simulink model "Four_DG_MG_PrimaryOnly"  (R2021b)
settings: Solver=ode23tb  StartTime=0.0  StopTime=5  RelTol=1e-3
model workspace (MAT data in the model file):
  Ts : Simulink.Parameter (value not decoded)
  secondary_on : Simulink.Parameter (value not decoded)
values from neighbouring files (symbols this model uses):
  a12 = 0    [Four_DG_MG_PrimaryOnlyScript.m]    (also in MPC_MG_script_raw_dmpc.m; MPC_MG_secondary_script.m)
  a14 = 0    [Four_DG_MG_PrimaryOnlyScript.m]    (also in MPC_MG_script_raw_dmpc.m; MPC_MG_secondary_script.m)
  a21 = 1    [Four_DG_MG_PrimaryOnlyScript.m]    (also in MPC_MG_script_raw_dmpc.m; MPC_MG_secondary_script.m)
  a23 = 0    [Four_DG_MG_PrimaryOnlyScript.m]    (also in MPC_MG_script_raw_dmpc.m; MPC_MG_secondary_script.m)
  a32 = 1    [Four_DG_MG_PrimaryOnlyScript.m]    (also in MPC_MG_script_raw_dmpc.m; MPC_MG_secondary_script.m)
  a34 = 0    [Four_DG_MG_PrimaryOnlyScript.m]    (also in MPC_MG_script_raw_dmpc.m; MPC_MG_secondary_script.m)
  a41 = 1    [Four_DG_MG_PrimaryOnlyScript.m]    (also in MPC_MG_script_raw_dmpc.m; MPC_MG_secondary_script.m)
  a43 = 0    [Four_DG_MG_PrimaryOnlyScript.m]    (also in MPC_MG_script_raw_dmpc.m; MPC_MG_secondary_script.m)
  b1v = 1    [Four_DG_MG_PrimaryOnlyScript.m]    (also in MPC_MG_script_raw_dmpc.m; MPC_MG_secondary_script.m; MPG_MG_July.m; MPG_MG_freq_script.m)
  b1w = 1    [Four_DG_MG_PrimaryOnlyScript.m]    (also in MPC_MG_script_raw_dmpc.m; MPC_MG_secondary_script.m; MPG_MG_July.m; MPG_MG_freq_script.m)
  b2v = 0    [Four_DG_MG_PrimaryOnlyScript.m]    (also in MPC_MG_script_raw_dmpc.m; MPC_MG_secondary_script.m; MPG_MG_July.m; MPG_MG_freq_script.m)
  b2w = 0    [Four_DG_MG_PrimaryOnlyScript.m]    (also in MPC_MG_script_raw_dmpc.m; MPC_MG_secondary_script.m; MPG_MG_July.m; MPG_MG_freq_script.m)
  b3v = 0    [Four_DG_MG_PrimaryOnlyScript.m]    (also in MPC_MG_script_raw_dmpc.m; MPC_MG_secondary_script.m; MPG_MG_July.m; MPG_MG_freq_script.m)
  b3w = 0    [Four_DG_MG_PrimaryOnlyScript.m]    (also in MPC_MG_script_raw_dmpc.m; MPC_MG_secondary_script.m; MPG_MG_July.m; MPG_MG_freq_script.m)
  b4v = 0    [Four_DG_MG_PrimaryOnlyScript.m]    (also in MPC_MG_script_raw_dmpc.m; MPC_MG_secondary_script.m; MPG_MG_July.m; MPG_MG_freq_script.m)
  b4w = 0    [Four_DG_MG_PrimaryOnlyScript.m]    (also in MPC_MG_script_raw_dmpc.m; MPC_MG_secondary_script.m; MPG_MG_July.m; MPG_MG_freq_script.m)
  C_f = 50e-6    (= 5e-05)    [Four_DG_MG_PrimaryOnlyScript.m]    (also in MPC_MG_script.m; MPC_MG_script_raw_dmpc.m; MPC_MG_secondary_script.m; MPG_MG_July.m)
  cf = 60    [Four_DG_MG_PrimaryOnlyScript.m]    (also in MPC_MG_script_raw_dmpc.m = 40; MPC_MG_secondary_script.m = 40; MPG_MG_July.m = 100; MPG_MG_freq_script.m = 100)
  cv = 60    [Four_DG_MG_PrimaryOnlyScript.m]    (also in MPC_MG_script_raw_dmpc.m = 40; MPC_MG_secondary_script.m = 40; MPG_MG_July.m = 100; MPG_MG_freq_script.m = 100)
  F = 1    [Four_DG_MG_PrimaryOnlyScript.m]    (also in dmpc.m = zeros(9,1))
  K_i1 = 420    [Four_DG_MG_PrimaryOnlyScript.m]
  K_i2 = K_i1    (= 420)    [Four_DG_MG_PrimaryOnlyScript.m]
  K_i3 = 390    [Four_DG_MG_PrimaryOnlyScript.m]
  K_i4 = K_i3    (= 390)    [Four_DG_MG_PrimaryOnlyScript.m]
  K_ii1 = 5e3    (= 5000)    [Four_DG_MG_PrimaryOnlyScript.m]
  K_ii2 = K_ii1    (= 5000)    [Four_DG_MG_PrimaryOnlyScript.m]
  K_ii3 = 16e3    (= 16000)    [Four_DG_MG_PrimaryOnlyScript.m]
  K_ii4 = K_ii3    (= 16000)    [Four_DG_MG_PrimaryOnlyScript.m]
  K_p1 = 0.1    [Four_DG_MG_PrimaryOnlyScript.m]
  K_p2 = K_p1    (= 0.1)    [Four_DG_MG_PrimaryOnlyScript.m]
  K_p3 = 0.05    [Four_DG_MG_PrimaryOnlyScript.m]
  K_p4 = K_p3    (= 0.05)    [Four_DG_MG_PrimaryOnlyScript.m]
  K_pi1 = 5    [Four_DG_MG_PrimaryOnlyScript.m]
  K_pi2 = K_pi1    (= 5)    [Four_DG_MG_PrimaryOnlyScript.m]
  K_pi3 = 10.5    [Four_DG_MG_PrimaryOnlyScript.m]
  K_pi4 = K_pi3    (= 10.5)    [Four_DG_MG_PrimaryOnlyScript.m]
  L_f = 1.35e-3    (= 0.00135)    [Four_DG_MG_PrimaryOnlyScript.m]    (also in MPC_MG_script.m; MPC_MG_script_raw_dmpc.m; MPC_MG_secondary_script.m; MPG_MG_July.m)
  L_in1 = 0.35e-3    (= 0.00035)    [Four_DG_MG_PrimaryOnlyScript.m]    (also in MPC_MG_script.m; MPC_MG_script_raw_dmpc.m; MPC_MG_secondary_script.m; MPG_MG_July.m)
  L_in2 = 0.35e-3    (= 0.00035)    [Four_DG_MG_PrimaryOnlyScript.m]    (also in MPC_MG_script.m; MPC_MG_script_raw_dmpc.m; MPC_MG_secondary_script.m; MPG_MG_July.m)
  L_in3 = 0.35e-3    (= 0.00035)    [Four_DG_MG_PrimaryOnlyScript.m]    (also in MPC_MG_script.m; MPC_MG_script_raw_dmpc.m; MPC_MG_secondary_script.m; MPG_MG_July.m)
  L_in4 = 0.35e-3    (= 0.00035)    [Four_DG_MG_PrimaryOnlyScript.m]    (also in MPC_MG_script.m; MPC_MG_script_raw_dmpc.m; MPC_MG_secondary_script.m; MPG_MG_July.m)
  lo_co = 0.2    [Four_DG_MG_PrimaryOnlyScript.m]    (also in MPC_MG_script.m = 0.05; MPC_MG_script_raw_dmpc.m; MPC_MG_secondary_script.m = 0.08; MPG_MG_July.m = 0.15)
  m_p1 = 9.4e-5/droopDivide    (= 9.4e-05)    [Four_DG_MG_PrimaryOnlyScript.m]    (also in MPC_MG_script.m; MPC_MG_script_raw_dmpc.m; MPC_MG_secondary_script.m; MPG_MG_July.m)
  m_p2 = 9.4e-5/droopDivide    (= 9.4e-05)    [Four_DG_MG_PrimaryOnlyScript.m]    (also in MPC_MG_script.m; MPC_MG_script_raw_dmpc.m; MPC_MG_secondary_script.m; MPG_MG_July.m)
  m_p3 = 12.5e-5/droopDivide    (= 0.000125)    [Four_DG_MG_PrimaryOnlyScript.m]    (also in MPC_MG_script.m; MPC_MG_script_raw_dmpc.m; MPC_MG_secondary_script.m; MPG_MG_July.m)
  m_p4 = 12.5e-5/droopDivide    (= 0.000125)    [Four_DG_MG_PrimaryOnlyScript.m]    (also in MPC_MG_script.m; MPC_MG_script_raw_dmpc.m; MPC_MG_secondary_script.m; MPG_MG_July.m)
  n_q1 = 1.3e-3/droopDivide2    (= 0.00013)    [Four_DG_MG_PrimaryOnlyScript.m]    (also in MPC_MG_script.m; MPC_MG_script_raw_dmpc.m; MPC_MG_secondary_script.m; MPG_MG_July.m)
  n_q2 = 1.3e-3/droopDivide2    (= 0.00013)    [Four_DG_MG_PrimaryOnlyScript.m]    (also in MPC_MG_script.m; MPC_MG_script_raw_dmpc.m; MPC_MG_secondary_script.m; MPG_MG_July.m)
  n_q3 = 1.5e-3/droopDivide2    (= 0.00015)    [Four_DG_MG_PrimaryOnlyScript.m]    (also in MPC_MG_script.m; MPC_MG_script_raw_dmpc.m; MPC_MG_secondary_script.m; MPG_MG_July.m)
  n_q4 = 1.5e-3/droopDivide2    (= 0.00015)    [Four_DG_MG_PrimaryOnlyScript.m]    (also in MPC_MG_script.m; MPC_MG_script_raw_dmpc.m; MPC_MG_secondary_script.m; MPG_MG_July.m)
  pq_gain = 3/2    (= 1.5)    [Four_DG_MG_PrimaryOnlyScript.m]
  R_f = 0.1    [Four_DG_MG_PrimaryOnlyScript.m]    (also in MPC_MG_script.m; MPC_MG_script_raw_dmpc.m; MPC_MG_secondary_script.m; MPG_MG_July.m)
  R_in1 = 0.03    [Four_DG_MG_PrimaryOnlyScript.m]    (also in MPC_MG_script.m; MPC_MG_script_raw_dmpc.m; MPC_MG_secondary_script.m; MPG_MG_July.m)
  R_in2 = 0.03    [Four_DG_MG_PrimaryOnlyScript.m]    (also in MPC_MG_script.m; MPC_MG_script_raw_dmpc.m; MPC_MG_secondary_script.m; MPG_MG_July.m)
  R_in3 = 0.03    [Four_DG_MG_PrimaryOnlyScript.m]    (also in MPC_MG_script.m; MPC_MG_script_raw_dmpc.m; MPC_MG_secondary_script.m; MPG_MG_July.m)
  R_in4 = 0.03    [Four_DG_MG_PrimaryOnlyScript.m]    (also in MPC_MG_script.m; MPC_MG_script_raw_dmpc.m; MPC_MG_secondary_script.m; MPG_MG_July.m)
  secondary = 1    [Four_DG_MG_PrimaryOnlyScript.m]
  secondary2 = 1    [Four_DG_MG_PrimaryOnlyScript.m]
  time_thresh = 0.6    [Four_DG_MG_PrimaryOnlyScript.m]    (also in MPC_MG_script_raw_dmpc.m = 1.5; MPC_MG_secondary_script.m = 2; MPG_MG_July.m = 0.5; MPG_MG_freq_script.m = 0.5)
  Ts = 10e-6    (= 1e-05)    [Four_DG_MG_PrimaryOnlyScript.m]    (also in MPC_MG_script.m; MPC_MG_script_raw_dmpc.m; MPC_MG_secondary_script.m; MPG_MG_July.m)
  V_nom = 220*sqrt(2)    [Four_DG_MG_PrimaryOnlyScript.m]    (also in MPC_MG_script.m; MPC_MG_script_raw_dmpc.m; MPC_MG_secondary_script.m; MPG_MG_July.m)
  Vdc = 600    [Four_DG_MG_PrimaryOnlyScript.m]    (also in MPC_MG_script.m; MPC_MG_script_raw_dmpc.m; MPC_MG_secondary_script.m; MPG_MG_July.m)
  w_nom = 2*pi*50    (= 314.159265359)    [Four_DG_MG_PrimaryOnlyScript.m]    (also in MPC_MG_script.m; MPC_MG_script_raw_dmpc.m; MPC_MG_secondary_script.m; MPG_MG_July.m)
undefined symbols (not defined in the file or in its folder): K_d
libraries: slpidlib x16, spsThreePhaseSeriesRLCBranchLib x15, spsabctodq0Lib x13, spsThreePhaseVIMeasurementLib x12, eeGeneralControl x8, spsOnDelayLib x8, spsPMUPLLBasedPositiveSequenceLib x4, eePwmGeneratorTwoLevel x4, spsdq0toabcLib x4, spsDCVoltageSourceLib x4, spsSeriesRLCBranchLib x4, spsTwoLevelConverterLib x4
(part 3 of 4)

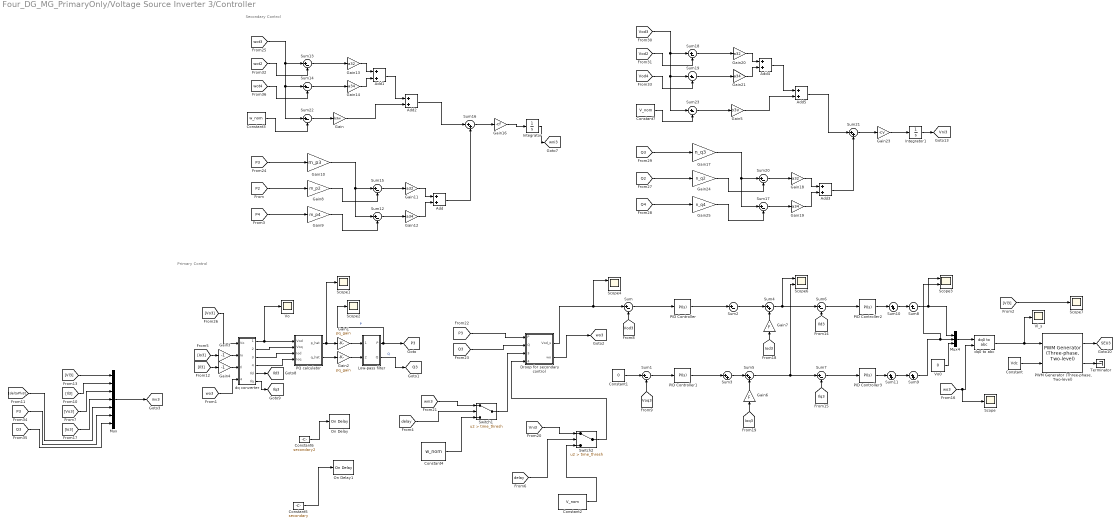
== system Four_DG_MG_PrimaryOnly/Voltage Source Inverter 3/Controller ==
  note: Secondary Control
  note: Primary Control
  Add{,1..5} (6 alike) : Sum
  Constant : Constant  Value=Vdc
  Constant1 : Constant  Value=0
  Constant2 : Constant  Value=V_nom
  Constant3 : Constant  Value=w_nom
  Constant4 : Constant  Value=w_nom
  Constant5 : Constant  Value=secondary
  Constant6 : Constant  Value=secondary2
  Constant7 : Constant  Value=V_nom
  Droop for secondary control : Subsystem
  Gain : Gain  Gain=b3w
  Gain1 : Gain  Gain=pq_gain
  Gain10 : Gain  Gain=m_p3
  Gain{11,13,18,20} (4 alike) : Gain  Gain=a32
  Gain{12,14,19,21} (4 alike) : Gain  Gain=a34
  Gain16 : Gain  Gain=-cf
  Gain17 : Gain  Gain=n_q3
  Gain2 : Gain  Gain=pq_gain
  Gain23 : Gain  Gain=-cv
  Gain24 : Gain  Gain=n_q2
  Gain25 : Gain  Gain=n_q4
  Gain3 : Gain  Gain=-1
  Gain4 : Gain  Gain=-1
  Gain5 : Gain  Gain=b3v
  Gain6 : Gain  Gain=F
  Gain7 : Gain  Gain=F
  Gain8 : Gain  Gain=m_p2
  Gain9 : Gain  Gain=m_p4
  Integrator : Integrator  InitialCondition=50*2*pi  UpperSaturationLimit=51*2*pi  LowerSaturationLimit=50*2*pi
  Integrator1 : Integrator  InitialCondition=311  UpperSaturationLimit=373.35  LowerSaturationLimit=248.90
  Low-pass filter : Subsystem
  Mux : Mux  Inputs=7
  Mux4 : Mux  Inputs=3
  On Delay : spsOnDelayLib/On Delay  DelayType=On delay  delay=4  ic=0  Ts=0
      settings: SourceProductBaseCode=PS
  On Delay1 : spsOnDelayLib/On Delay  DelayType=On delay  delay=4  ic=0  Ts=0
      settings: SourceProductBaseCode=PS
  PID Controller : slpidlib/PID Controller  Controller=PI  Form=Parallel  TimeDomain=Continuous-time  UseExternalTs=off  SampleTime=-1  IntegratorMethod=Forward Euler  FilterMethod=Forward Euler  ControllerParametersSource=internal  P=K_p3  I=K_i3  D=K_d  UseFilter=on  N=100  TunerSelectOption=Frequency Response Based  InitialConditionSource=internal  InitialConditionForIntegrator=0  InitialConditionForFilter=0  DifferentiatorICPrevScaledInput=0  ExternalReset=none  TrackingMode=off  Kt=1  LimitOutput=off  SatLimitsSource=internal  UpperSaturationLimit=50  LowerSaturationLimit=-50  LinearizeAsGain=on  AntiWindupMode=none  Kb=1  POutMin=[]  POutMax=[]  IOutMin=[]  IOutMax=[]  DOutMin=[]  DOutMax=[]  NOutMin=[]  NOutMax=[]  SumOutMin=[]  SumOutMax=[]  SaturationOutMin=[]  SaturationOutMax=[]  PParamMin=[]  PParamMax=[]  IParamMin=[]  IParamMax=[]  DParamMin=[]  DParamMax=[]  NParamMin=[]  NParamMax=[]  KbParamMin=[]  KbParamMax=[]  KtParamMin=[]  KtParamMax=[]  KbOutMin=[]  KbOutMax=[]  KtOutMin=[]  KtOutMax=[]  IntegratorOutMin=[]  IntegratorOutMax=[]  FilterOutMin=[]  FilterOutMax=[]  SumI1OutMin=[]  SumI1OutMax=[]  SumI2OutMin=[]  SumI2OutMax=[]  SumI3OutMin=[]  SumI3OutMax=[]  SumI4OutMin=[]  SumI4OutMax=[]  SumDOutMin=[]  SumDOutMax=[]  DifferentiatorOutMin=[]  DifferentiatorOutMax=[]  FilterDiffOutCoefMin=[]  FilterDiffOutCoefMax=[]  ReciprocalOutMin=[]  ReciprocalOutMax=[]  SumDenOutMin=[]  SumDenOutMax=[]  SumNumOutMin=[]  SumNumOutMax=[]  DivideOutMin=[]  DivideOutMax=[]  UdiffTsProdOutMin=[]  UdiffTsProdOutMax=[]  NTsProdOutMin=[]  NTsProdOutMax=[]  UintegralTsProdOutMin=[]  UintegralTsProdOutMax=[]  UngainTsProdOutMin=[]  UngainTsProdOutMax=[]  IntegratorContinuousStateAttributes=''  IntegratorStateMustResolveToSignalObject=off  IntegratorRTWStateStorageClass=Auto  FilterContinuousStateAttributes=''  FilterStateMustResolveToSignalObject=off  FilterRTWStateStorageClass=Auto  ParallelPVariant=InternalParameters  IdealPVariant=Disabled  IVariant=InternalParameters  DVariant=Disabled  IntegratorVariant=Continuous  SatVariant=Disabled  AWVariant=Passthrough  PCopyVariant=Disabled  TRVariant=Disabled  FdbkBlocksVariant=Forward  IdealPFdbkVariant=Disabled  SatFdbkVariant=Disabled  DerivativeFilterVariant=Disabled  NVariant=Disabled  NCopyVariant=Disabled_SignalSpec  FilterICVariant=Disabled  IntegratorICVariant=InternalICs  ExternalResetVariant=Disabled  TRSumVariant=Passthrough  SumFdbkVariant=Disabled  SumVariant=Sum_PI  TsampFilterVariant=InternalTs  TsampNgainVariant=Passthrough  TsampIntegralVariant=Passthrough  ExternalSaturationOutDataTypeStr=Inherit: Same as second input
  PID Controller1 : slpidlib/PID Controller  Controller=PI  Form=Parallel  TimeDomain=Continuous-time  UseExternalTs=off  SampleTime=-1  IntegratorMethod=Forward Euler  FilterMethod=Forward Euler  ControllerParametersSource=internal  P=K_p3  I=K_i3  D=K_d  UseFilter=on  N=100  TunerSelectOption=Frequency Response Based  InitialConditionSource=internal  InitialConditionForIntegrator=0  InitialConditionForFilter=0  DifferentiatorICPrevScaledInput=0  ExternalReset=none  TrackingMode=off  Kt=1  LimitOutput=off  SatLimitsSource=internal  UpperSaturationLimit=50  LowerSaturationLimit=-50  LinearizeAsGain=on  AntiWindupMode=none  Kb=1  POutMin=[]  POutMax=[]  IOutMin=[]  IOutMax=[]  DOutMin=[]  DOutMax=[]  NOutMin=[]  NOutMax=[]  SumOutMin=[]  SumOutMax=[]  SaturationOutMin=[]  SaturationOutMax=[]  PParamMin=[]  PParamMax=[]  IParamMin=[]  IParamMax=[]  DParamMin=[]  DParamMax=[]  NParamMin=[]  NParamMax=[]  KbParamMin=[]  KbParamMax=[]  KtParamMin=[]  KtParamMax=[]  KbOutMin=[]  KbOutMax=[]  KtOutMin=[]  KtOutMax=[]  IntegratorOutMin=[]  IntegratorOutMax=[]  FilterOutMin=[]  FilterOutMax=[]  SumI1OutMin=[]  SumI1OutMax=[]  SumI2OutMin=[]  SumI2OutMax=[]  SumI3OutMin=[]  SumI3OutMax=[]  SumI4OutMin=[]  SumI4OutMax=[]  SumDOutMin=[]  SumDOutMax=[]  DifferentiatorOutMin=[]  DifferentiatorOutMax=[]  FilterDiffOutCoefMin=[]  FilterDiffOutCoefMax=[]  ReciprocalOutMin=[]  ReciprocalOutMax=[]  SumDenOutMin=[]  SumDenOutMax=[]  SumNumOutMin=[]  SumNumOutMax=[]  DivideOutMin=[]  DivideOutMax=[]  UdiffTsProdOutMin=[]  UdiffTsProdOutMax=[]  NTsProdOutMin=[]  NTsProdOutMax=[]  UintegralTsProdOutMin=[]  UintegralTsProdOutMax=[]  UngainTsProdOutMin=[]  UngainTsProdOutMax=[]  IntegratorContinuousStateAttributes=''  IntegratorStateMustResolveToSignalObject=off  IntegratorRTWStateStorageClass=Auto  FilterContinuousStateAttributes=''  FilterStateMustResolveToSignalObject=off  FilterRTWStateStorageClass=Auto  ParallelPVariant=InternalParameters  IdealPVariant=Disabled  IVariant=InternalParameters  DVariant=Disabled  IntegratorVariant=Continuous  SatVariant=Disabled  AWVariant=Passthrough  PCopyVariant=Disabled  TRVariant=Disabled  FdbkBlocksVariant=Forward  IdealPFdbkVariant=Disabled  SatFdbkVariant=Disabled  DerivativeFilterVariant=Disabled  NVariant=Disabled  NCopyVariant=Disabled_SignalSpec  FilterICVariant=Disabled  IntegratorICVariant=InternalICs  ExternalResetVariant=Disabled  TRSumVariant=Passthrough  SumFdbkVariant=Disabled  SumVariant=Sum_PI  TsampFilterVariant=InternalTs  TsampNgainVariant=Passthrough  TsampIntegralVariant=Passthrough  ExternalSaturationOutDataTypeStr=Inherit: Same as second input
  PID Controller2 : slpidlib/PID Controller  Controller=PI  Form=Parallel  TimeDomain=Continuous-time  UseExternalTs=off  SampleTime=-1  IntegratorMethod=Forward Euler  FilterMethod=Forward Euler  ControllerParametersSource=internal  P=K_pi3  I=K_ii3  D=K_d  UseFilter=on  N=100  TunerSelectOption=Frequency Response Based  InitialConditionSource=internal  InitialConditionForIntegrator=0  InitialConditionForFilter=0  DifferentiatorICPrevScaledInput=0  ExternalReset=none  TrackingMode=off  Kt=1  LimitOutput=off  SatLimitsSource=internal  UpperSaturationLimit=inf  LowerSaturationLimit=-inf  LinearizeAsGain=on  AntiWindupMode=none  Kb=1  POutMin=[]  POutMax=[]  IOutMin=[]  IOutMax=[]  DOutMin=[]  DOutMax=[]  NOutMin=[]  NOutMax=[]  SumOutMin=[]  SumOutMax=[]  SaturationOutMin=[]  SaturationOutMax=[]  PParamMin=[]  PParamMax=[]  IParamMin=[]  IParamMax=[]  DParamMin=[]  DParamMax=[]  NParamMin=[]  NParamMax=[]  KbParamMin=[]  KbParamMax=[]  KtParamMin=[]  KtParamMax=[]  KbOutMin=[]  KbOutMax=[]  KtOutMin=[]  KtOutMax=[]  IntegratorOutMin=[]  IntegratorOutMax=[]  FilterOutMin=[]  FilterOutMax=[]  SumI1OutMin=[]  SumI1OutMax=[]  SumI2OutMin=[]  SumI2OutMax=[]  SumI3OutMin=[]  SumI3OutMax=[]  SumI4OutMin=[]  SumI4OutMax=[]  SumDOutMin=[]  SumDOutMax=[]  DifferentiatorOutMin=[]  DifferentiatorOutMax=[]  FilterDiffOutCoefMin=[]  FilterDiffOutCoefMax=[]  ReciprocalOutMin=[]  ReciprocalOutMax=[]  SumDenOutMin=[]  SumDenOutMax=[]  SumNumOutMin=[]  SumNumOutMax=[]  DivideOutMin=[]  DivideOutMax=[]  UdiffTsProdOutMin=[]  UdiffTsProdOutMax=[]  NTsProdOutMin=[]  NTsProdOutMax=[]  UintegralTsProdOutMin=[]  UintegralTsProdOutMax=[]  UngainTsProdOutMin=[]  UngainTsProdOutMax=[]  IntegratorContinuousStateAttributes=''  IntegratorStateMustResolveToSignalObject=off  IntegratorRTWStateStorageClass=Auto  FilterContinuousStateAttributes=''  FilterStateMustResolveToSignalObject=off  FilterRTWStateStorageClass=Auto  ParallelPVariant=InternalParameters  IdealPVariant=Disabled  IVariant=InternalParameters  DVariant=Disabled  IntegratorVariant=Continuous  SatVariant=Disabled  AWVariant=Passthrough  PCopyVariant=Disabled  TRVariant=Disabled  FdbkBlocksVariant=Forward  IdealPFdbkVariant=Disabled  SatFdbkVariant=Disabled  DerivativeFilterVariant=Disabled  NVariant=Disabled  NCopyVariant=Disabled_SignalSpec  FilterICVariant=Disabled  IntegratorICVariant=InternalICs  ExternalResetVariant=Disabled  TRSumVariant=Passthrough  SumFdbkVariant=Disabled  SumVariant=Sum_PI  TsampFilterVariant=InternalTs  TsampNgainVariant=Passthrough  TsampIntegralVariant=Passthrough  ExternalSaturationOutDataTypeStr=Inherit: Same as second input
  PID Controller3 : slpidlib/PID Controller  Controller=PI  Form=Parallel  TimeDomain=Continuous-time  UseExternalTs=off  SampleTime=-1  IntegratorMethod=Forward Euler  FilterMethod=Forward Euler  ControllerParametersSource=internal  P=K_pi3  I=K_ii3  D=K_d  UseFilter=on  N=100  TunerSelectOption=Frequency Response Based  InitialConditionSource=internal  InitialConditionForIntegrator=0  InitialConditionForFilter=0  DifferentiatorICPrevScaledInput=0  ExternalReset=none  TrackingMode=off  Kt=1  LimitOutput=off  SatLimitsSource=internal  UpperSaturationLimit=inf  LowerSaturationLimit=-inf  LinearizeAsGain=on  AntiWindupMode=none  Kb=1  POutMin=[]  POutMax=[]  IOutMin=[]  IOutMax=[]  DOutMin=[]  DOutMax=[]  NOutMin=[]  NOutMax=[]  SumOutMin=[]  SumOutMax=[]  SaturationOutMin=[]  SaturationOutMax=[]  PParamMin=[]  PParamMax=[]  IParamMin=[]  IParamMax=[]  DParamMin=[]  DParamMax=[]  NParamMin=[]  NParamMax=[]  KbParamMin=[]  KbParamMax=[]  KtParamMin=[]  KtParamMax=[]  KbOutMin=[]  KbOutMax=[]  KtOutMin=[]  KtOutMax=[]  IntegratorOutMin=[]  IntegratorOutMax=[]  FilterOutMin=[]  FilterOutMax=[]  SumI1OutMin=[]  SumI1OutMax=[]  SumI2OutMin=[]  SumI2OutMax=[]  SumI3OutMin=[]  SumI3OutMax=[]  SumI4OutMin=[]  SumI4OutMax=[]  SumDOutMin=[]  SumDOutMax=[]  DifferentiatorOutMin=[]  DifferentiatorOutMax=[]  FilterDiffOutCoefMin=[]  FilterDiffOutCoefMax=[]  ReciprocalOutMin=[]  ReciprocalOutMax=[]  SumDenOutMin=[]  SumDenOutMax=[]  SumNumOutMin=[]  SumNumOutMax=[]  DivideOutMin=[]  DivideOutMax=[]  UdiffTsProdOutMin=[]  UdiffTsProdOutMax=[]  NTsProdOutMin=[]  NTsProdOutMax=[]  UintegralTsProdOutMin=[]  UintegralTsProdOutMax=[]  UngainTsProdOutMin=[]  UngainTsProdOutMax=[]  IntegratorContinuousStateAttributes=''  IntegratorStateMustResolveToSignalObject=off  IntegratorRTWStateStorageClass=Auto  FilterContinuousStateAttributes=''  FilterStateMustResolveToSignalObject=off  FilterRTWStateStorageClass=Auto  ParallelPVariant=InternalParameters  IdealPVariant=Disabled  IVariant=InternalParameters  DVariant=Disabled  IntegratorVariant=Continuous  SatVariant=Disabled  AWVariant=Passthrough  PCopyVariant=Disabled  TRVariant=Disabled  FdbkBlocksVariant=Forward  IdealPFdbkVariant=Disabled  SatFdbkVariant=Disabled  DerivativeFilterVariant=Disabled  NVariant=Disabled  NCopyVariant=Disabled_SignalSpec  FilterICVariant=Disabled  IntegratorICVariant=InternalICs  ExternalResetVariant=Disabled  TRSumVariant=Passthrough  SumFdbkVariant=Disabled  SumVariant=Sum_PI  TsampFilterVariant=InternalTs  TsampNgainVariant=Passthrough  TsampIntegralVariant=Passthrough  ExternalSaturationOutDataTypeStr=Inherit: Same as second input
  PQ calculator : Subsystem
  "PWM Generator (Three-phase, Two-level)" : eePwmGeneratorTwoLevel/PWM Generator (Three-phase, Two-level)  PWMMode=Continuous PWM (CPWM)  CPWMMode=SPWM: sinusoidal PWM  DPWMMode=60 DPWM: 60 degree discontinuous PWM  fsw=f_c  Ts=Ts
      settings: SourceProductBaseCode=PS
  Scope{,1..2,7} (4 alike) : Scope
  Scope3 : Scope  NumInputPorts=2
  Scope4 : Scope  NumInputPorts=2
  Scope6 : Scope  NumInputPorts=2
  Sum{,1..2,6..8,12..15,17..20,22..23} (16 alike) : Sum  Inputs=|+-
  Sum{3..5,9..11,16,21} (8 alike) : Sum  Inputs=|++
  Switch1 : Switch  Criteria=u2 > Threshold  Threshold=time_thresh
  Switch2 : Switch  Criteria=u2 > Threshold  Threshold=time_thresh
  Terminator : Terminator
  Vl_s : Scope
  Vo : Scope
  Vo0 : Constant  Value=0
  dq converter : Subsystem
  dq0 to abc : spsdq0toabcLib/dq0 to abc  Alignment=90 degrees behind phase A axis
  tag scope: Ild3=global, Ilq3=global, P3=global, Q3=global, SEU3=global, Vni3=global, inv3=global, wni3=global, wo3=global
  wires:
  dq converter/1(Vod) -> Vo/1, PQ calculator/1(Vod)
  ? -> Sum3/2
  [Vl3] -> Scope7/1
  [Io3] -> Gain3/1
  Sum/1 -> PID Controller/1
  dq converter/6(Ilq) -> [Ilq3]
  Sum1/1 -> PID Controller1/1
  Sum7/1 -> PID Controller3/1
  [Voq3] -> Sum1/2
  dq converter/5(Ild) -> [Ild3]
  Mux4/1 -> dq0 to abc/1
  PID Controller/1 -> Sum2/1
  PID Controller1/1 -> Sum3/1
  Vo0/1 -> Mux4/3
  Sum6/1 -> PID Controller2/1
  Sum2/1 -> Sum4/1
  PQ calculator/1(p_hat) -> Gain1/1, Scope1/1
  [Il3] -> Gain4/1
  [Vo3] -> dq converter/1(Vo)
  Sum9/1 -> Scope3/2, Mux4/2
  Gain6/1 -> Sum5/2
  dq converter/4(Ioq) -> PQ calculator/4(Ioq)
  "PWM Generator (Three-phase, Two-level)"/2 -> Terminator/1
  Sum5/1 -> Scope6/2, Sum7/1
  Constant/1 -> "PWM Generator (Three-phase, Two-level)"/2
  dq converter/3(Iod) -> PQ calculator/3(Iod)
  dq converter/2(Voq) -> PQ calculator/2(Voq)
  Sum8/1 -> Scope3/1, Mux4/1
  [Ioq3] -> Gain6/1
  dq0 to abc/1 -> Vl_s/1, "PWM Generator (Three-phase, Two-level)"/1
  [Ilq3] -> Sum7/2
  Gain1/1 -> Low-pass filter/1(p_hat)
  "PWM Generator (Three-phase, Two-level)"/1 -> [SEU3]
  [Ild3] -> Sum6/2
  [Vod3] -> Sum/2
  PQ calculator/2(q_hat) -> Gain2/1
  Low-pass filter/1(P) -> [P3], Scope2/1  "P"
  Droop for secondary control/2(wo) -> [wo3]
  [Q3] -> Droop for secondary control/2(Q)
  [P3] -> Droop for secondary control/1(P)
  Gain7/1 -> Sum4/2
  [Iod3] -> Gain7/1
  Sum4/1 -> Scope6/1, Sum6/1
  Sum3/1 -> Sum5/1
  Gain2/1 -> Low-pass filter/2(q_hat)
  Low-pass filter/2(Q) -> [Q3]  "Q"
  [wni3] -> Switch1/1
  Constant4/1 -> Switch1/3
  Switch1/1 -> Droop for secondary control/3(w_nom)
  Switch2/1 -> Droop for secondary control/4(V_nom)
  [Vni3] -> Switch2/1
  Constant2/1 -> Switch2/3
  [wo3] -> Scope/1, dq0 to abc/2
  [wo3] -> dq converter/4(wo3)
  Droop for secondary control/1(Vod_s) -> Scope4/1, Sum/1
  PID Controller3/1 -> Sum11/1
  Sum11/1 -> Sum9/1
  PID Controller2/1 -> Sum10/1
  Sum10/1 -> Sum8/1
  Constant1/1 -> Sum1/1
  Gain3/1 -> dq converter/2(Io)
  Gain4/1 -> dq converter/3(Il)
  Sum16/1 -> Gain16/1
  [Q2] -> Gain24/1
  Gain10/1 -> Sum12/1, Sum15/1
  Sum14/1 -> Gain14/1
  [wot2] -> Sum13/2
  Integrator/1 -> [wni3]
  Gain13/1 -> Add1/1
  Gain19/1 -> Add3/2
  [Vod4] -> Sum19/2
  Sum17/1 -> Gain19/1
  [Q3] -> Gain17/1
  Sum21/1 -> Gain23/1
  [Vod3] -> Sum23/1, Sum19/1, Sum18/1
  Gain9/1 -> Sum12/2
  Gain24/1 -> Sum20/2
  Gain11/1 -> Add/1
  [P4] -> Gain9/1
  Sum13/1 -> Gain13/1
  Sum20/1 -> Gain18/1
  [Q4] -> Gain25/1
  Sum12/1 -> Gain12/1
  Gain16/1 -> Integrator/1
  Gain8/1 -> Sum15/2
  Gain25/1 -> Sum17/2
  Sum15/1 -> Gain11/1
  Add3/1 -> Sum21/2
  Gain14/1 -> Add1/2
  Sum19/1 -> Gain21/1
  [wot4] -> Sum14/2
  Gain21/1 -> Add4/2
  Add/1 -> Sum16/2
  [wot3] -> Sum22/1, Sum14/1, Sum13/1
  [Vod2] -> Sum18/2
  Gain20/1 -> Add4/1
  Integrator1/1 -> [Vni3]
  Gain12/1 -> Add/2
  Gain18/1 -> Add3/1
  Sum18/1 -> Gain20/1
  Gain17/1 -> Sum17/1, Sum20/1
  [P3] -> Gain10/1
  Gain23/1 -> Integrator1/1
  [P2] -> Gain8/1
  Constant6/1 -> On Delay/1
  Constant5/1 -> On Delay1/1
  [delay] -> Switch1/2
  [delay] -> Switch2/2
  Constant3/1 -> Sum22/2
  Sum22/1 -> Gain/1
  Add1/1 -> Add2/1
  Gain/1 -> Add2/2
  Add2/1 -> Sum16/1
  Constant7/1 -> Sum23/2
  Sum23/1 -> Gain5/1
  Add4/1 -> Add5/1
  Gain5/1 -> Add5/2
  Add5/1 -> Sum21/1
  [Vo3] -> Mux/3
  [P3] -> Mux/6
  [deltaPhi3] -> Mux/5
  [Vl3] -> Mux/1
  Mux/1 -> [inv3]
  [Q3] -> Mux/7
  [Il3] -> Mux/2
  [Io3] -> Mux/4

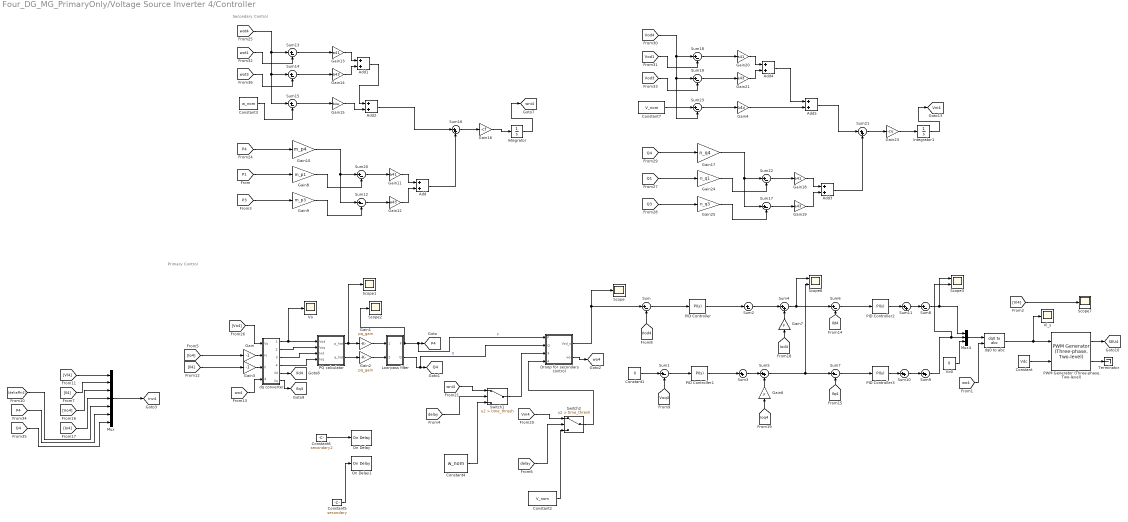
== system Four_DG_MG_PrimaryOnly/Voltage Source Inverter 4/Controller ==
  note: Secondary Control
  note: Primary Control
  Add{,1..5} (6 alike) : Sum
  Constant : Constant  Value=Vdc
  Constant1 : Constant  Value=0
  Constant2 : Constant  Value=V_nom
  Constant3 : Constant  Value=w_nom
  Constant4 : Constant  Value=w_nom
  Constant5 : Constant  Value=secondary
  Constant6 : Constant  Value=secondary2
  Constant7 : Constant  Value=V_nom
  Droop for secondary control : Subsystem
  Gain : Gain  Gain=-1
  Gain1 : Gain  Gain=pq_gain
  Gain10 : Gain  Gain=m_p4
  Gain{11,13,18,20} (4 alike) : Gain  Gain=a41
  Gain{12,14,19,21} (4 alike) : Gain  Gain=a43
  Gain15 : Gain  Gain=b4w
  Gain16 : Gain  Gain=-cf
  Gain17 : Gain  Gain=n_q4
  Gain2 : Gain  Gain=pq_gain
  Gain23 : Gain  Gain=-cv
  Gain24 : Gain  Gain=n_q1
  Gain25 : Gain  Gain=n_q3
  Gain3 : Gain  Gain=-1
  Gain4 : Gain  Gain=b4v
  Gain6 : Gain  Gain=F
  Gain7 : Gain  Gain=F
  Gain8 : Gain  Gain=m_p1
  Gain9 : Gain  Gain=m_p3
  Integrator : Integrator  InitialCondition=50*2*pi  UpperSaturationLimit=51*2*pi  LowerSaturationLimit=50*2*pi
  Integrator1 : Integrator  InitialCondition=311  UpperSaturationLimit=373.35  LowerSaturationLimit=248.90
  Low-pass filter : Subsystem
  Mux : Mux  Inputs=7
  Mux4 : Mux  Inputs=3
  On Delay : spsOnDelayLib/On Delay  DelayType=On delay  delay=4  ic=0  Ts=0
      settings: SourceProductBaseCode=PS
  On Delay1 : spsOnDelayLib/On Delay  DelayType=On delay  delay=4  ic=0  Ts=0
      settings: SourceProductBaseCode=PS
  PID Controller : slpidlib/PID Controller  Controller=PI  Form=Parallel  TimeDomain=Continuous-time  UseExternalTs=off  SampleTime=-1  IntegratorMethod=Forward Euler  FilterMethod=Forward Euler  ControllerParametersSource=internal  P=K_p4  I=K_i4  D=K_d  UseFilter=on  N=100  TunerSelectOption=Frequency Response Based  InitialConditionSource=internal  InitialConditionForIntegrator=0  InitialConditionForFilter=0  DifferentiatorICPrevScaledInput=0  ExternalReset=none  TrackingMode=off  Kt=1  LimitOutput=off  SatLimitsSource=internal  UpperSaturationLimit=50  LowerSaturationLimit=-50  LinearizeAsGain=on  AntiWindupMode=none  Kb=1  POutMin=[]  POutMax=[]  IOutMin=[]  IOutMax=[]  DOutMin=[]  DOutMax=[]  NOutMin=[]  NOutMax=[]  SumOutMin=[]  SumOutMax=[]  SaturationOutMin=[]  SaturationOutMax=[]  PParamMin=[]  PParamMax=[]  IParamMin=[]  IParamMax=[]  DParamMin=[]  DParamMax=[]  NParamMin=[]  NParamMax=[]  KbParamMin=[]  KbParamMax=[]  KtParamMin=[]  KtParamMax=[]  KbOutMin=[]  KbOutMax=[]  KtOutMin=[]  KtOutMax=[]  IntegratorOutMin=[]  IntegratorOutMax=[]  FilterOutMin=[]  FilterOutMax=[]  SumI1OutMin=[]  SumI1OutMax=[]  SumI2OutMin=[]  SumI2OutMax=[]  SumI3OutMin=[]  SumI3OutMax=[]  SumI4OutMin=[]  SumI4OutMax=[]  SumDOutMin=[]  SumDOutMax=[]  DifferentiatorOutMin=[]  DifferentiatorOutMax=[]  FilterDiffOutCoefMin=[]  FilterDiffOutCoefMax=[]  ReciprocalOutMin=[]  ReciprocalOutMax=[]  SumDenOutMin=[]  SumDenOutMax=[]  SumNumOutMin=[]  SumNumOutMax=[]  DivideOutMin=[]  DivideOutMax=[]  UdiffTsProdOutMin=[]  UdiffTsProdOutMax=[]  NTsProdOutMin=[]  NTsProdOutMax=[]  UintegralTsProdOutMin=[]  UintegralTsProdOutMax=[]  UngainTsProdOutMin=[]  UngainTsProdOutMax=[]  IntegratorContinuousStateAttributes=''  IntegratorStateMustResolveToSignalObject=off  IntegratorRTWStateStorageClass=Auto  FilterContinuousStateAttributes=''  FilterStateMustResolveToSignalObject=off  FilterRTWStateStorageClass=Auto  ParallelPVariant=InternalParameters  IdealPVariant=Disabled  IVariant=InternalParameters  DVariant=Disabled  IntegratorVariant=Continuous  SatVariant=Disabled  AWVariant=Passthrough  PCopyVariant=Disabled  TRVariant=Disabled  FdbkBlocksVariant=Forward  IdealPFdbkVariant=Disabled  SatFdbkVariant=Disabled  DerivativeFilterVariant=Disabled  NVariant=Disabled  NCopyVariant=Disabled_SignalSpec  FilterICVariant=Disabled  IntegratorICVariant=InternalICs  ExternalResetVariant=Disabled  TRSumVariant=Passthrough  SumFdbkVariant=Disabled  SumVariant=Sum_PI  TsampFilterVariant=InternalTs  TsampNgainVariant=Passthrough  TsampIntegralVariant=Passthrough  ExternalSaturationOutDataTypeStr=Inherit: Same as second input
  PID Controller1 : slpidlib/PID Controller  Controller=PI  Form=Parallel  TimeDomain=Continuous-time  UseExternalTs=off  SampleTime=-1  IntegratorMethod=Forward Euler  FilterMethod=Forward Euler  ControllerParametersSource=internal  P=K_p4  I=K_i4  D=K_d  UseFilter=on  N=100  TunerSelectOption=Frequency Response Based  InitialConditionSource=internal  InitialConditionForIntegrator=0  InitialConditionForFilter=0  DifferentiatorICPrevScaledInput=0  ExternalReset=none  TrackingMode=off  Kt=1  LimitOutput=off  SatLimitsSource=internal  UpperSaturationLimit=50  LowerSaturationLimit=-50  LinearizeAsGain=on  AntiWindupMode=none  Kb=1  POutMin=[]  POutMax=[]  IOutMin=[]  IOutMax=[]  DOutMin=[]  DOutMax=[]  NOutMin=[]  NOutMax=[]  SumOutMin=[]  SumOutMax=[]  SaturationOutMin=[]  SaturationOutMax=[]  PParamMin=[]  PParamMax=[]  IParamMin=[]  IParamMax=[]  DParamMin=[]  DParamMax=[]  NParamMin=[]  NParamMax=[]  KbParamMin=[]  KbParamMax=[]  KtParamMin=[]  KtParamMax=[]  KbOutMin=[]  KbOutMax=[]  KtOutMin=[]  KtOutMax=[]  IntegratorOutMin=[]  IntegratorOutMax=[]  FilterOutMin=[]  FilterOutMax=[]  SumI1OutMin=[]  SumI1OutMax=[]  SumI2OutMin=[]  SumI2OutMax=[]  SumI3OutMin=[]  SumI3OutMax=[]  SumI4OutMin=[]  SumI4OutMax=[]  SumDOutMin=[]  SumDOutMax=[]  DifferentiatorOutMin=[]  DifferentiatorOutMax=[]  FilterDiffOutCoefMin=[]  FilterDiffOutCoefMax=[]  ReciprocalOutMin=[]  ReciprocalOutMax=[]  SumDenOutMin=[]  SumDenOutMax=[]  SumNumOutMin=[]  SumNumOutMax=[]  DivideOutMin=[]  DivideOutMax=[]  UdiffTsProdOutMin=[]  UdiffTsProdOutMax=[]  NTsProdOutMin=[]  NTsProdOutMax=[]  UintegralTsProdOutMin=[]  UintegralTsProdOutMax=[]  UngainTsProdOutMin=[]  UngainTsProdOutMax=[]  IntegratorContinuousStateAttributes=''  IntegratorStateMustResolveToSignalObject=off  IntegratorRTWStateStorageClass=Auto  FilterContinuousStateAttributes=''  FilterStateMustResolveToSignalObject=off  FilterRTWStateStorageClass=Auto  ParallelPVariant=InternalParameters  IdealPVariant=Disabled  IVariant=InternalParameters  DVariant=Disabled  IntegratorVariant=Continuous  SatVariant=Disabled  AWVariant=Passthrough  PCopyVariant=Disabled  TRVariant=Disabled  FdbkBlocksVariant=Forward  IdealPFdbkVariant=Disabled  SatFdbkVariant=Disabled  DerivativeFilterVariant=Disabled  NVariant=Disabled  NCopyVariant=Disabled_SignalSpec  FilterICVariant=Disabled  IntegratorICVariant=InternalICs  ExternalResetVariant=Disabled  TRSumVariant=Passthrough  SumFdbkVariant=Disabled  SumVariant=Sum_PI  TsampFilterVariant=InternalTs  TsampNgainVariant=Passthrough  TsampIntegralVariant=Passthrough  ExternalSaturationOutDataTypeStr=Inherit: Same as second input
  PID Controller2 : slpidlib/PID Controller  Controller=PI  Form=Parallel  TimeDomain=Continuous-time  UseExternalTs=off  SampleTime=-1  IntegratorMethod=Forward Euler  FilterMethod=Forward Euler  ControllerParametersSource=internal  P=K_pi4  I=K_ii4  D=K_d  UseFilter=on  N=100  TunerSelectOption=Frequency Response Based  InitialConditionSource=internal  InitialConditionForIntegrator=0  InitialConditionForFilter=0  DifferentiatorICPrevScaledInput=0  ExternalReset=none  TrackingMode=off  Kt=1  LimitOutput=off  SatLimitsSource=internal  UpperSaturationLimit=inf  LowerSaturationLimit=-inf  LinearizeAsGain=on  AntiWindupMode=none  Kb=1  POutMin=[]  POutMax=[]  IOutMin=[]  IOutMax=[]  DOutMin=[]  DOutMax=[]  NOutMin=[]  NOutMax=[]  SumOutMin=[]  SumOutMax=[]  SaturationOutMin=[]  SaturationOutMax=[]  PParamMin=[]  PParamMax=[]  IParamMin=[]  IParamMax=[]  DParamMin=[]  DParamMax=[]  NParamMin=[]  NParamMax=[]  KbParamMin=[]  KbParamMax=[]  KtParamMin=[]  KtParamMax=[]  KbOutMin=[]  KbOutMax=[]  KtOutMin=[]  KtOutMax=[]  IntegratorOutMin=[]  IntegratorOutMax=[]  FilterOutMin=[]  FilterOutMax=[]  SumI1OutMin=[]  SumI1OutMax=[]  SumI2OutMin=[]  SumI2OutMax=[]  SumI3OutMin=[]  SumI3OutMax=[]  SumI4OutMin=[]  SumI4OutMax=[]  SumDOutMin=[]  SumDOutMax=[]  DifferentiatorOutMin=[]  DifferentiatorOutMax=[]  FilterDiffOutCoefMin=[]  FilterDiffOutCoefMax=[]  ReciprocalOutMin=[]  ReciprocalOutMax=[]  SumDenOutMin=[]  SumDenOutMax=[]  SumNumOutMin=[]  SumNumOutMax=[]  DivideOutMin=[]  DivideOutMax=[]  UdiffTsProdOutMin=[]  UdiffTsProdOutMax=[]  NTsProdOutMin=[]  NTsProdOutMax=[]  UintegralTsProdOutMin=[]  UintegralTsProdOutMax=[]  UngainTsProdOutMin=[]  UngainTsProdOutMax=[]  IntegratorContinuousStateAttributes=''  IntegratorStateMustResolveToSignalObject=off  IntegratorRTWStateStorageClass=Auto  FilterContinuousStateAttributes=''  FilterStateMustResolveToSignalObject=off  FilterRTWStateStorageClass=Auto  ParallelPVariant=InternalParameters  IdealPVariant=Disabled  IVariant=InternalParameters  DVariant=Disabled  IntegratorVariant=Continuous  SatVariant=Disabled  AWVariant=Passthrough  PCopyVariant=Disabled  TRVariant=Disabled  FdbkBlocksVariant=Forward  IdealPFdbkVariant=Disabled  SatFdbkVariant=Disabled  DerivativeFilterVariant=Disabled  NVariant=Disabled  NCopyVariant=Disabled_SignalSpec  FilterICVariant=Disabled  IntegratorICVariant=InternalICs  ExternalResetVariant=Disabled  TRSumVariant=Passthrough  SumFdbkVariant=Disabled  SumVariant=Sum_PI  TsampFilterVariant=InternalTs  TsampNgainVariant=Passthrough  TsampIntegralVariant=Passthrough  ExternalSaturationOutDataTypeStr=Inherit: Same as second input
  PID Controller3 : slpidlib/PID Controller  Controller=PI  Form=Parallel  TimeDomain=Continuous-time  UseExternalTs=off  SampleTime=-1  IntegratorMethod=Forward Euler  FilterMethod=Forward Euler  ControllerParametersSource=internal  P=K_pi4  I=K_ii4  D=K_d  UseFilter=on  N=100  TunerSelectOption=Frequency Response Based  InitialConditionSource=internal  InitialConditionForIntegrator=0  InitialConditionForFilter=0  DifferentiatorICPrevScaledInput=0  ExternalReset=none  TrackingMode=off  Kt=1  LimitOutput=off  SatLimitsSource=internal  UpperSaturationLimit=inf  LowerSaturationLimit=-inf  LinearizeAsGain=on  AntiWindupMode=none  Kb=1  POutMin=[]  POutMax=[]  IOutMin=[]  IOutMax=[]  DOutMin=[]  DOutMax=[]  NOutMin=[]  NOutMax=[]  SumOutMin=[]  SumOutMax=[]  SaturationOutMin=[]  SaturationOutMax=[]  PParamMin=[]  PParamMax=[]  IParamMin=[]  IParamMax=[]  DParamMin=[]  DParamMax=[]  NParamMin=[]  NParamMax=[]  KbParamMin=[]  KbParamMax=[]  KtParamMin=[]  KtParamMax=[]  KbOutMin=[]  KbOutMax=[]  KtOutMin=[]  KtOutMax=[]  IntegratorOutMin=[]  IntegratorOutMax=[]  FilterOutMin=[]  FilterOutMax=[]  SumI1OutMin=[]  SumI1OutMax=[]  SumI2OutMin=[]  SumI2OutMax=[]  SumI3OutMin=[]  SumI3OutMax=[]  SumI4OutMin=[]  SumI4OutMax=[]  SumDOutMin=[]  SumDOutMax=[]  DifferentiatorOutMin=[]  DifferentiatorOutMax=[]  FilterDiffOutCoefMin=[]  FilterDiffOutCoefMax=[]  ReciprocalOutMin=[]  ReciprocalOutMax=[]  SumDenOutMin=[]  SumDenOutMax=[]  SumNumOutMin=[]  SumNumOutMax=[]  DivideOutMin=[]  DivideOutMax=[]  UdiffTsProdOutMin=[]  UdiffTsProdOutMax=[]  NTsProdOutMin=[]  NTsProdOutMax=[]  UintegralTsProdOutMin=[]  UintegralTsProdOutMax=[]  UngainTsProdOutMin=[]  UngainTsProdOutMax=[]  IntegratorContinuousStateAttributes=''  IntegratorStateMustResolveToSignalObject=off  IntegratorRTWStateStorageClass=Auto  FilterContinuousStateAttributes=''  FilterStateMustResolveToSignalObject=off  FilterRTWStateStorageClass=Auto  ParallelPVariant=InternalParameters  IdealPVariant=Disabled  IVariant=InternalParameters  DVariant=Disabled  IntegratorVariant=Continuous  SatVariant=Disabled  AWVariant=Passthrough  PCopyVariant=Disabled  TRVariant=Disabled  FdbkBlocksVariant=Forward  IdealPFdbkVariant=Disabled  SatFdbkVariant=Disabled  DerivativeFilterVariant=Disabled  NVariant=Disabled  NCopyVariant=Disabled_SignalSpec  FilterICVariant=Disabled  IntegratorICVariant=InternalICs  ExternalResetVariant=Disabled  TRSumVariant=Passthrough  SumFdbkVariant=Disabled  SumVariant=Sum_PI  TsampFilterVariant=InternalTs  TsampNgainVariant=Passthrough  TsampIntegralVariant=Passthrough  ExternalSaturationOutDataTypeStr=Inherit: Same as second input
  PQ calculator : Subsystem
  "PWM Generator (Three-phase, Two-level)" : eePwmGeneratorTwoLevel/PWM Generator (Three-phase, Two-level)  PWMMode=Continuous PWM (CPWM)  CPWMMode=SPWM: sinusoidal PWM  DPWMMode=60 DPWM: 60 degree discontinuous PWM  fsw=f_c  Ts=Ts
      settings: SourceProductBaseCode=PS
  Scope{,1..2,7} (4 alike) : Scope
  Scope3 : Scope  NumInputPorts=2
  Scope6 : Scope  NumInputPorts=2
  Sum{,1..2,6..8,12..15,17..20,22..23} (16 alike) : Sum  Inputs=|+-
  Sum{3..5,9..11,16,21} (8 alike) : Sum  Inputs=|++
  Switch1 : Switch  Criteria=u2 > Threshold  Threshold=time_thresh
  Switch2 : Switch  Criteria=u2 > Threshold  Threshold=time_thresh
  Terminator : Terminator
  Vl_s : Scope
  Vo : Scope
  Vo0 : Constant  Value=0
  dq converter : Subsystem
  dq0 to abc : spsdq0toabcLib/dq0 to abc  Alignment=90 degrees behind phase A axis
  tag scope: Ild4=global, Ilq4=global, P4=global, Q4=global, SEU4=global, Vni4=global, inv4=global, wni4=global, wo4=global
  wires:
  dq converter/1(Vod) -> Vo/1, PQ calculator/1(Vod)
  [Vl4] -> Scope7/1
  [Io4] -> Gain/1
  Sum/1 -> PID Controller/1
  dq converter/6(Ilq) -> [Ilq4]
  Sum1/1 -> PID Controller1/1
  Sum7/1 -> PID Controller3/1
  [Voq4] -> Sum1/2
  dq converter/5(Ild) -> [Ild4]
  Mux4/1 -> dq0 to abc/1
  PID Controller/1 -> Sum2/1
  PID Controller1/1 -> Sum3/1
  Vo0/1 -> Mux4/3
  Sum6/1 -> PID Controller2/1
  Sum2/1 -> Sum4/1
  PQ calculator/1(p_hat) -> Gain1/1, Scope1/1
  [Il4] -> Gain3/1
  [Vo4] -> dq converter/1(Vo)
  Sum9/1 -> Scope3/2, Mux4/2
  Gain6/1 -> Sum5/2
  dq converter/4(Ioq) -> PQ calculator/4(Ioq)
  "PWM Generator (Three-phase, Two-level)"/2 -> Terminator/1
  Sum5/1 -> Sum7/1, Scope6/2
  Constant/1 -> "PWM Generator (Three-phase, Two-level)"/2
  dq converter/3(Iod) -> PQ calculator/3(Iod)
  dq converter/2(Voq) -> PQ calculator/2(Voq)
  Sum8/1 -> Scope3/1, Mux4/1
  [Ioq4] -> Gain6/1
  dq0 to abc/1 -> Vl_s/1, "PWM Generator (Three-phase, Two-level)"/1
  [Ilq4] -> Sum7/2
  Gain1/1 -> Low-pass filter/1(p_hat)
  "PWM Generator (Three-phase, Two-level)"/1 -> [SEU4]
  [Ild4] -> Sum6/2
  [Vod4] -> Sum/2
  PQ calculator/2(q_hat) -> Gain2/1
  Low-pass filter/1(P) -> Droop for secondary control/1(P), [P4], Scope2/1  "P"
  Gain7/1 -> Sum4/2
  [Iod4] -> Gain7/1
  Sum4/1 -> Sum6/1, Scope6/1
  Sum3/1 -> Sum5/1
  Gain2/1 -> Low-pass filter/2(q_hat)
  Low-pass filter/2(Q) -> Droop for secondary control/2(Q), [Q4]  "Q"
  Switch1/1 -> Droop for secondary control/3(w_nom)
  [wni4] -> Switch1/1
  Constant4/1 -> Switch1/3
  Switch2/1 -> Droop for secondary control/4(V_nom)
  [Vni4] -> Switch2/1
  Constant2/1 -> Switch2/3
  [wo4] -> dq0 to abc/2
  ? -> Sum3/2
  [wo4] -> dq converter/4(wo4)
  Droop for secondary control/1(Vod_s) -> Sum/1, Scope/1
  Droop for secondary control/2(wo) -> [wo4]
  PID Controller3/1 -> Sum10/1
  Sum10/1 -> Sum9/1
  PID Controller2/1 -> Sum11/1
  Sum11/1 -> Sum8/1
  Constant1/1 -> Sum1/1
  Gain/1 -> dq converter/2(Io)
  Gain3/1 -> dq converter/3(Il)
  Add2/1 -> Sum16/1
  Sum18/1 -> Gain20/1
  Gain16/1 -> Integrator/1
  Sum16/1 -> Gain16/1
  Gain23/1 -> Integrator1/1
  Sum21/1 -> Gain23/1
  Gain9/1 -> Sum12/2
  [Q1] -> Gain24/1
  [Vod3] -> Sum19/2
  Gain10/1 -> Sum12/1, Sum20/1
  Sum22/1 -> Gain18/1
  Gain25/1 -> Sum17/2
  [Vod1] -> Sum18/2
  Add3/1 -> Sum21/2
  Add1/1 -> Add2/1
  Gain12/1 -> Add/2
  [Q3] -> Gain25/1
  [P3] -> Gain9/1
  [wot3] -> Sum14/2
  Gain19/1 -> Add3/2
  [wot1] -> Sum13/2
  Sum14/1 -> Gain14/1
  Integrator/1 -> [wni4]
  Sum15/1 -> Gain15/1
  Sum13/1 -> Gain13/1
  Add/1 -> Sum16/2
  Gain24/1 -> Sum22/2
  Gain13/1 -> Add1/1
  Sum19/1 -> Gain21/1
  [wot4] -> Sum15/1, Sum14/1, Sum13/1
  Sum20/1 -> Gain11/1
  Sum12/1 -> Gain12/1
  Gain21/1 -> Add4/2
  Sum17/1 -> Gain19/1
  [P4] -> Gain10/1
  Gain20/1 -> Add4/1
  Constant3/1 -> Sum15/2
  Gain15/1 -> Add2/2
  Gain8/1 -> Sum20/2
  Gain11/1 -> Add/1
  Integrator1/1 -> [Vni4]
  Gain14/1 -> Add1/2
  [Vod4] -> Sum23/2, Sum19/1, Sum18/1
  [Q4] -> Gain17/1
  [P1] -> Gain8/1
  Gain17/1 -> Sum17/1, Sum22/1
  Gain18/1 -> Add3/1
  Constant6/1 -> On Delay/1
  Constant5/1 -> On Delay1/1
  [delay] -> Switch1/2
  [delay] -> Switch2/2
  Constant7/1 -> Sum23/1
  Sum23/1 -> Gain4/1
  Gain4/1 -> Add5/2
  Add4/1 -> Add5/1
  Add5/1 -> Sum21/1
  [Vo4] -> Mux/3
  [P4] -> Mux/6
  [deltaPhi4] -> Mux/5
  [Vl4] -> Mux/1
  Mux/1 -> [inv4]
  [Q4] -> Mux/7
  [Il4] -> Mux/2
  [Io4] -> Mux/4

== system Four_DG_MG_PrimaryOnly/Voltage Source Inverter 1/Controller/Droop for secondary control ==
  P : Inport
  Q : Inport  Port=2
  w_nom : Inport  Port=3
  V_nom : Inport  Port=4
  Gain4 : Gain  Gain=n_q1
  Gain5 : Gain  Gain=m_p1
  Integrator : Integrator  WrapState=on  WrappedStateUpperValue=2*pi  WrappedStateLowerValue=0
  Sum1 : Sum  Inputs=|+-
  Sum2 : Sum  Inputs=|+-
  Vod_s : Outport
  wo : Outport  Port=2
  tag scope: wot1=global
  wires:
  P/1 -> Gain5/1
  V_nom/1 -> Sum1/1
  Q/1 -> Gain4/1
  w_nom/1 -> Sum2/1
  Gain5/1 -> Sum2/2
  Gain4/1 -> Sum1/2
  Sum2/1 -> [wot1], Integrator/1  "w"
  Integrator/1 -> wo/1
  Sum1/1 -> Vod_s/1  "Vod_s"

== system Four_DG_MG_PrimaryOnly/Voltage Source Inverter 1/Controller/Low-pass filter ==
  p_hat : Inport
  q_hat : Inport  Port=2
  Low-Pass Filter (Discrete or Continuous) : eeGeneralControl/Low-Pass Filter (Discrete or Continuous)  K=1  T=lo_co  B=inf  A=-inf  init_option=Inherited from block input  x0=0  Ts=-1
  Low-Pass Filter (Discrete or Continuous)1 : eeGeneralControl/Low-Pass Filter (Discrete or Continuous)  K=1  T=lo_co  B=inf  A=-inf  init_option=Inherited from block input  x0=0  Ts=-1
  P : Outport
  Q : Outport  Port=2
  wires:
  q_hat/1 -> Low-Pass Filter (Discrete or Continuous)1/1
  Low-Pass Filter (Discrete or Continuous)1/1 -> Q/1  "Q"
  Low-Pass Filter (Discrete or Continuous)/1 -> P/1  "P"
  p_hat/1 -> Low-Pass Filter (Discrete or Continuous)/1

== system Four_DG_MG_PrimaryOnly/Voltage Source Inverter 1/Controller/PQ calculator ==
  Vod : Inport
  Voq : Inport  Port=2
  Iod : Inport  Port=3
  Ioq : Inport  Port=4
  Product{,1..3} (4 alike) : Product
  Sum10 : Sum  Inputs=|++
  Sum11 : Sum  Inputs=|+-
  p_hat : Outport
  q_hat : Outport  Port=2
  wires:
  Product3/1 -> Sum11/2
  Product1/1 -> Sum10/2
  Voq/1 -> Product3/1, Product1/1
  Iod/1 -> Product/2, Product3/2
  Product2/1 -> Sum11/1
  Ioq/1 -> Product1/2, Product2/2
  Product/1 -> Sum10/1
  Vod/1 -> Product/1, Product2/1
  Sum11/1 -> q_hat/1  "q_hat"
  Sum10/1 -> p_hat/1  "p_hat"

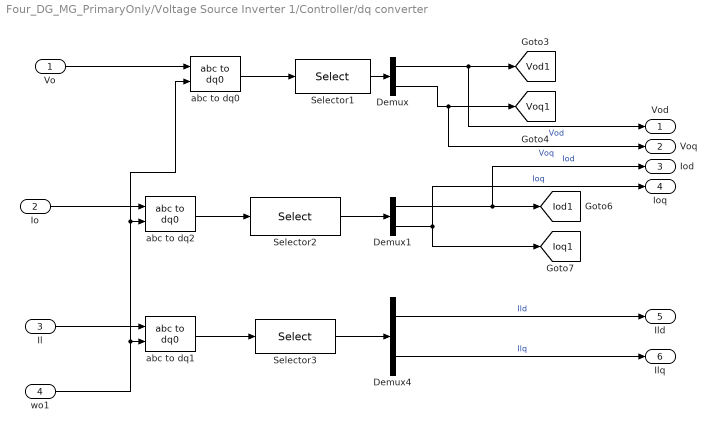
== system Four_DG_MG_PrimaryOnly/Voltage Source Inverter 1/Controller/dq converter ==
  Vo : Inport
  Io : Inport  Port=2
  Il : Inport  Port=3
  wo1 : Inport  Port=4
  Demux : Demux  Outputs=2
  Demux1 : Demux  Outputs=2
  Demux4 : Demux  Outputs=2
  Selector1 : Selector  InputPortWidth=3  IndexOptions=Index vector (dialog)  Indices=[1 2]  OutputSizes=1
  Selector2 : Selector  InputPortWidth=3  IndexOptions=Index vector (dialog)  Indices=[1 2]  OutputSizes=1
  Selector3 : Selector  InputPortWidth=3  IndexOptions=Index vector (dialog)  Indices=[1 2]  OutputSizes=1
  abc to dq0 : spsabctodq0Lib/abc to dq0  Alignment=90 degrees behind phase A axis
  abc to dq1 : spsabctodq0Lib/abc to dq0  Alignment=90 degrees behind phase A axis
  abc to dq2 : spsabctodq0Lib/abc to dq0  Alignment=90 degrees behind phase A axis
  Vod : Outport
  Voq : Outport  Port=2
  Iod : Outport  Port=3
  Ioq : Outport  Port=4
  Ild : Outport  Port=5
  Ilq : Outport  Port=6
  tag scope: Iod1=global, Ioq1=global, Vod1=global, Voq1=global
  wires:
  Vo/1 -> abc to dq0/1
  Demux/1 -> Vod/1, [Vod1]  "Vod"
  Demux1/1 -> Iod/1, [Iod1]  "Iod"
  wo1/1 -> abc to dq0/2, abc to dq2/2, abc to dq1/2
  Selector3/1 -> Demux4/1
  Demux/2 -> Voq/1, [Voq1]  "Voq"
  Selector1/1 -> Demux/1
  abc to dq2/1 -> Selector2/1
  abc to dq1/1 -> Selector3/1
  Demux1/2 -> Ioq/1, [Ioq1]  "Ioq"
  Demux4/1 -> Ild/1  "Ild"
  abc to dq0/1 -> Selector1/1
  Selector2/1 -> Demux1/1
  Io/1 -> abc to dq2/1
  Il/1 -> abc to dq1/1
  Demux4/2 -> Ilq/1  "Ilq"

== system Four_DG_MG_PrimaryOnly/Voltage Source Inverter 2/Controller/Droop for secondary control ==
  P : Inport
  Q : Inport  Port=2
  w_nom : Inport  Port=3
  V_nom : Inport  Port=4
  Gain4 : Gain  Gain=n_q2
  Gain5 : Gain  Gain=m_p2
  Integrator : Integrator  WrapState=on  WrappedStateUpperValue=2*pi  WrappedStateLowerValue=0
  Sum1 : Sum  Inputs=|+-
  Sum2 : Sum  Inputs=|+-
  Vod_s : Outport
  wo : Outport  Port=2
  tag scope: wot2=global
  wires:
  P/1 -> Gain5/1
  V_nom/1 -> Sum1/1
  Q/1 -> Gain4/1
  w_nom/1 -> Sum2/1
  Gain5/1 -> Sum2/2
  Gain4/1 -> Sum1/2
  Sum2/1 -> [wot2], Integrator/1  "w"
  Integrator/1 -> wo/1
  Sum1/1 -> Vod_s/1  "Vod_s"

== system Four_DG_MG_PrimaryOnly/Voltage Source Inverter 2/Controller/Low-pass filter ==
  p_hat : Inport
  q_hat : Inport  Port=2
  Low-Pass Filter (Discrete or Continuous) : eeGeneralControl/Low-Pass Filter (Discrete or Continuous)  K=1  T=lo_co  B=inf  A=-inf  init_option=Inherited from block input  x0=0  Ts=-1
  Low-Pass Filter (Discrete or Continuous)1 : eeGeneralControl/Low-Pass Filter (Discrete or Continuous)  K=1  T=lo_co  B=inf  A=-inf  init_option=Inherited from block input  x0=0  Ts=-1
  P : Outport
  Q : Outport  Port=2
  wires:
  q_hat/1 -> Low-Pass Filter (Discrete or Continuous)1/1
  Low-Pass Filter (Discrete or Continuous)1/1 -> Q/1  "Q"
  Low-Pass Filter (Discrete or Continuous)/1 -> P/1  "P"
  p_hat/1 -> Low-Pass Filter (Discrete or Continuous)/1

== system Four_DG_MG_PrimaryOnly/Voltage Source Inverter 2/Controller/PQ calculator ==
  Vod : Inport
  Voq : Inport  Port=2
  Iod : Inport  Port=3
  Ioq : Inport  Port=4
  Product{,1..3} (4 alike) : Product
  Sum10 : Sum  Inputs=|++
  Sum11 : Sum  Inputs=|+-
  p_hat : Outport
  q_hat : Outport  Port=2
  wires:
  Product3/1 -> Sum11/2
  Product1/1 -> Sum10/2
  Voq/1 -> Product3/1, Product1/1
  Iod/1 -> Product/2, Product3/2
  Product2/1 -> Sum11/1
  Ioq/1 -> Product1/2, Product2/2
  Product/1 -> Sum10/1
  Vod/1 -> Product/1, Product2/1
  Sum11/1 -> q_hat/1  "q_hat"
  Sum10/1 -> p_hat/1  "p_hat"

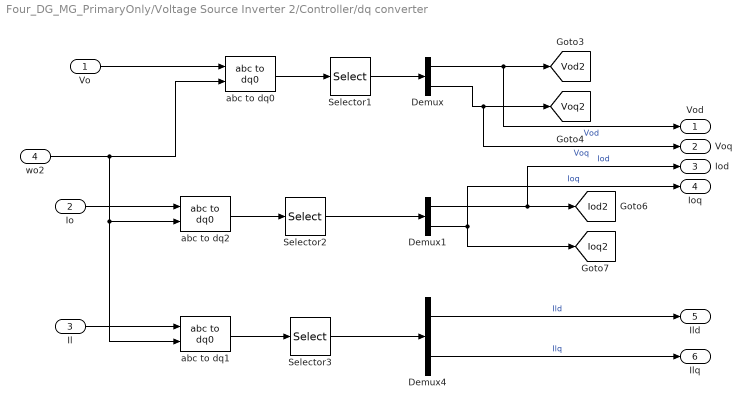
== system Four_DG_MG_PrimaryOnly/Voltage Source Inverter 2/Controller/dq converter ==
  Vo : Inport
  Io : Inport  Port=2
  Il : Inport  Port=3
  wo2 : Inport  Port=4
  Demux : Demux  Outputs=2
  Demux1 : Demux  Outputs=2
  Demux4 : Demux  Outputs=2
  Selector1 : Selector  InputPortWidth=3  IndexOptions=Index vector (dialog)  Indices=[1 2]  OutputSizes=1
  Selector2 : Selector  InputPortWidth=3  IndexOptions=Index vector (dialog)  Indices=[1 2]  OutputSizes=1
  Selector3 : Selector  InputPortWidth=3  IndexOptions=Index vector (dialog)  Indices=[1 2]  OutputSizes=1
  abc to dq0 : spsabctodq0Lib/abc to dq0  Alignment=90 degrees behind phase A axis
  abc to dq1 : spsabctodq0Lib/abc to dq0  Alignment=90 degrees behind phase A axis
  abc to dq2 : spsabctodq0Lib/abc to dq0  Alignment=90 degrees behind phase A axis
  Vod : Outport
  Voq : Outport  Port=2
  Iod : Outport  Port=3
  Ioq : Outport  Port=4
  Ild : Outport  Port=5
  Ilq : Outport  Port=6
  tag scope: Iod2=global, Ioq2=global, Vod2=global, Voq2=global
  wires:
  Vo/1 -> abc to dq0/1
  Demux/1 -> Vod/1, [Vod2]  "Vod"
  Demux1/1 -> Iod/1, [Iod2]  "Iod"
  Selector3/1 -> Demux4/1
  Demux/2 -> Voq/1, [Voq2]  "Voq"
  Selector1/1 -> Demux/1
  abc to dq2/1 -> Selector2/1
  abc to dq1/1 -> Selector3/1
  wo2/1 -> abc to dq1/2, abc to dq2/2, abc to dq0/2
  Demux1/2 -> Ioq/1, [Ioq2]  "Ioq"
  Demux4/1 -> Ild/1  "Ild"
  abc to dq0/1 -> Selector1/1
  Selector2/1 -> Demux1/1
  Io/1 -> abc to dq2/1
  Il/1 -> abc to dq1/1
  Demux4/2 -> Ilq/1  "Ilq"

== system Four_DG_MG_PrimaryOnly/Voltage Source Inverter 3/Controller/Droop for secondary control ==
  P : Inport
  Q : Inport  Port=2
  w_nom : Inport  Port=3
  V_nom : Inport  Port=4
  Gain4 : Gain  Gain=n_q3
  Gain5 : Gain  Gain=m_p3
  Integrator : Integrator  WrapState=on  WrappedStateUpperValue=2*pi  WrappedStateLowerValue=0
  Sum1 : Sum  Inputs=|+-
  Sum2 : Sum  Inputs=|+-
  Vod_s : Outport
  wo : Outport  Port=2
  tag scope: wot3=global
  wires:
  P/1 -> Gain5/1
  V_nom/1 -> Sum1/1
  Q/1 -> Gain4/1
  w_nom/1 -> Sum2/1
  Gain5/1 -> Sum2/2
  Gain4/1 -> Sum1/2
  Sum2/1 -> [wot3], Integrator/1  "w"
  Integrator/1 -> wo/1
  Sum1/1 -> Vod_s/1  "Vod_s"

== system Four_DG_MG_PrimaryOnly/Voltage Source Inverter 3/Controller/Low-pass filter ==
  p_hat : Inport
  q_hat : Inport  Port=2
  Low-Pass Filter (Discrete or Continuous) : eeGeneralControl/Low-Pass Filter (Discrete or Continuous)  K=1  T=lo_co  B=inf  A=-inf  init_option=Inherited from block input  x0=0  Ts=-1
  Low-Pass Filter (Discrete or Continuous)1 : eeGeneralControl/Low-Pass Filter (Discrete or Continuous)  K=1  T=lo_co  B=inf  A=-inf  init_option=Inherited from block input  x0=0  Ts=-1
  P : Outport
  Q : Outport  Port=2
  wires:
  q_hat/1 -> Low-Pass Filter (Discrete or Continuous)1/1
  Low-Pass Filter (Discrete or Continuous)1/1 -> Q/1  "Q"
  Low-Pass Filter (Discrete or Continuous)/1 -> P/1  "P"
  p_hat/1 -> Low-Pass Filter (Discrete or Continuous)/1
